simulink model "exportarC_digo"  (R2025b)
settings: Solver=FixedStepAuto  StartTime=0.0  StopTime=149.86  FixedStep=0.1  MaxStep=0.1  RelTol=1e-3
model workspace (MAT data in the model file):
  Sig = Simulink.Signal
  Sig.Dimensions = -1
  Sig.DimensionsMode = 'auto'
  Sig.Complexity = 'auto'
  Sig.SampleTime = -1
  Sig.SamplingMode = 'auto'
  Sig.DataType = 'auto'
libraries: cstblocks x1, mpclib x1
settings Model: PauseTimes=4  Creator=mulusoy  LastModifiedBy=gabcc
settings OptimizationCC: DefaultParameterBehavior=Inlined  EnhancedBackFolding=on  PassReuseOutputArgsAs=Individual arguments  ZeroExternalMemoryAtStartup=off  ZeroInternalMemoryAtStartup=off  OptimizeBlockOrder=speed  DifferentSizesBufferReuse=on  OptimizationCustomize=off  EfficientTunableParamExpr=on
settings DebuggingCC: ParameterTunabilityLossMsg=error
settings HardwareCC: ProdBitPerPointer=32.0  ProdBitPerSizeT=32.0  ProdBitPerPtrDiffT=32.0  ProdLargestAtomicFloat=None  ProdWordSize=32.0  ProdHWDeviceType=Custom Processor->Custom Processor
settings SFSimCC: MATLABDynamicMemAlloc=off
settings RTWCC: SystemTargetFile=ert.tlc  TemplateMakefile=ert_default_tmf  TargetLang=C++  GPUComputeCapability=3.5  Description=Embedded Coder
settings CodeAppCC: ForceParamTrailComments=on  IgnoreCustomStorageClasses=off  OperatorAnnotations=on  SimulinkDataObjDesc=on  SFDataObjDesc=on  InsertBlockDesc=on
settings ERTTargetCC: RootIOFormat=Structure reference  ERTCustomFileTemplate=example_file_process.tlc  TargetLangStandard=C++11 (ISO)  GenerateSampleERTMain=on  CodeInterfacePackaging=C++ class  SubcomponentCodeInterfacePackaging=C++ class

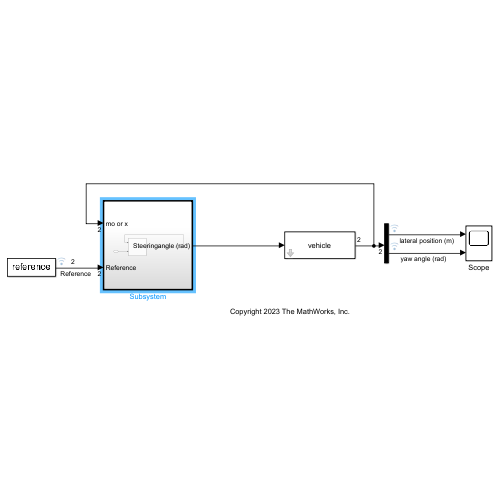
[thumbnail: Simulink's stored preview of the top-level diagram]
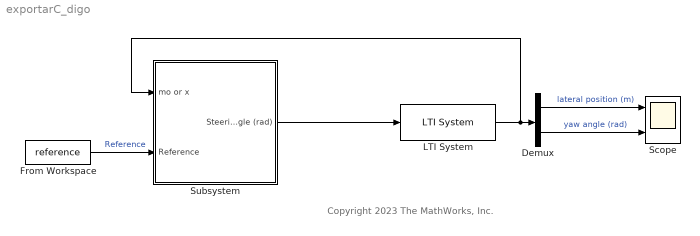
== system exportarC_digo ==
  note: Copyright 2023 The MathWorks, Inc.
  Demux : Demux  Outputs=2
  From Workspace : FromWorkspace  VariableName=reference
  LTI System : cstblocks/LTI System  sys=vehicle  IC=[]  PadeOrder=0
  Scope : Scope  NumInputPorts=2
      settings: ActiveDisplayYMinimum=-38.531562903984536  ActiveDisplayYMaximum=43.24337062360209  DataLoggingVariableName=simout
  Subsystem : Subsystem  TreatAsAtomicUnit=on
  wires:
  LTI System/1 -> Subsystem/1(mo or x), Demux/1
  Demux/1 -> Scope/1  "lateral position (m)"
  Demux/2 -> Scope/2  "yaw angle (rad)"
  From Workspace/1 -> Subsystem/2(Reference)  "Reference"
  Subsystem/1(Steeringangle (rad)) -> LTI System/1

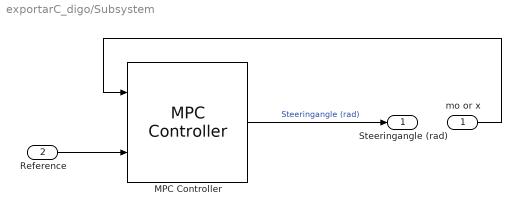
== system exportarC_digo/Subsystem ==
  mo or x : Inport
  Reference : Inport  Port=2
  MPC Controller : mpclib/MPC Controller  SCDEnableBlockLinearizationSpecification=on  mpcobj=mpc1  is_multiple=0  enable_value=0  return_u0=off  updateMPCinCallerWorkspace=on  md_inport=off  mv_inport=off  uref_inport=off  return_cost=off  return_mvseq=off  return_qpstatus=off  return_xseq=off  return_state=off  return_ovseq=off  state_inport=off  umin_inport=off  umax_inport=off  ymin_inport=off  ymax_inport=off  cc_inport=off  ywt_inport=off  uwt_inport=off  duwt_inport=off  rhoeps_inport=off  pm_inport=off  MaximumP=10  HorizonChoice=FixedHorizon  n_ts=0.1  n_p=15  n_mv=1  n_md=0  n_ud=0  n_mo=2  n_uo=0  BlockDataType=double  SampleTimeInherited=off  switch_inport=off
  Steeringangle (rad) : Outport
  wires:
  mo or x/1 -> MPC Controller/1
  Reference/1 -> MPC Controller/2
  MPC Controller/1 -> Steeringangle (rad)/1  "Steeringangle (rad)"
